simulink model "PositionControl"  (R2023a)
settings: Solver=FixedStepAuto  StartTime=0.0  StopTime=100.0  FixedStep=Ts  RelTol=1e-3
values from neighbouring files (symbols this model uses):
  refx = 5    [generar_circuito.m]    (also in generar_trayectoria.m = 1.3236)
  refy = 0    [generar_circuito.m]    (also in generar_trayectoria.m = -4.0246)
undefined symbols (not defined in the file or in its folder): DiscIntNeverNeededParam
libraries: fuzblock x1
settings Model: PacingRate=100  Creator=mfran  LastModifiedBy=mfran
settings DataIOCC: ReturnWorkspaceOutputs=off

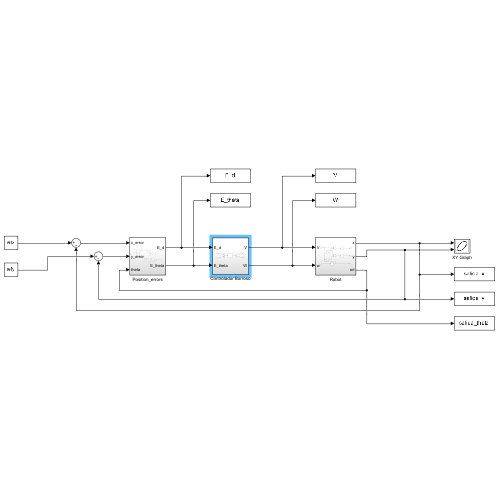
[thumbnail: Simulink's stored preview of the top-level diagram]
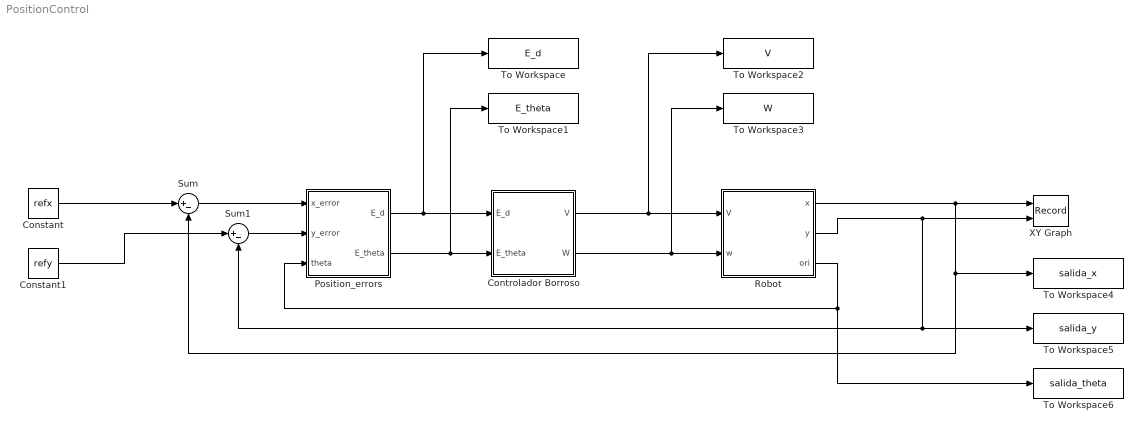
== system PositionControl ==
  Constant : Constant  Value=refx
  Constant1 : Constant  Value=refy
  Controlador Borroso : Subsystem
  Position_errors : Subsystem
  Robot : Subsystem
  Sum : Sum  Inputs=|+-
  Sum1 : Sum  Inputs=|+-
  To Workspace : ToWorkspace  VariableName=E_d  SaveFormat=Timeseries  SampleTime=-1
  To Workspace1 : ToWorkspace  VariableName=E_theta  SaveFormat=Timeseries  SampleTime=-1
  To Workspace2 : ToWorkspace  VariableName=V  SaveFormat=Timeseries  SampleTime=-1
  To Workspace3 : ToWorkspace  VariableName=W  SaveFormat=Timeseries  SampleTime=-1
  To Workspace4 : ToWorkspace  VariableName=salida_x  SaveFormat=Timeseries  SampleTime=-1
  To Workspace5 : ToWorkspace  VariableName=salida_y  SaveFormat=Timeseries  SampleTime=-1
  To Workspace6 : ToWorkspace  VariableName=salida_theta  SaveFormat=Timeseries  SampleTime=-1
  XY Graph : Record  FileSettingsInternal="{\"entries\":[{\"content\":{\"excelSettings\":{\"content\":{},\"type\":\"Streamout.ExcelSettings\"}},\"type\":\"Streamout.FileSettingStorage\",\"uuid\":\"\"}],\"packageUris\":[\"http:\\/\\/schema.mathworks.com\\/mf0\\/streamout_blocks\\/R2020a\"],\"version\":\"1.0\"}"  Layout=[1 1]  SignalsInternal="{\"entries\":[{\"content\":{\"signals\":[{\"content\":{\"blockPath\":[],\"dimensions\":[1],\"domain\":\"\",\"lineColor\":\"#a2142f\",\"plots\":[1],\"port\":1,\"sid\":[\"\"],\"signalID\":8169,\"signalName\":\"Robot:1\"},\"type\":\"RecordBlkView.Signal\",\"uuid\":\"\"},{\"content\":{\"blockPath\":[],\"dimensions\":[1],\"domain\":\"\",\"lineColor\":\"#139fff\",\"plots\":[1],\"port\":2,\"sid\":[\"\"],\"signalID\":8173,\"signalName\":\"Robot:2\"},\"type\":\"RecordBlkView.Signal\",\"uuid\":\"\"}]},\"type\":\"RecordBlkView.InputSignals\",\"uuid\":\"\"}],\"packageUris\":[\"http:\\/\\/schema.mathworks.com\\/mf0\\/streamout_blocks\\/R2020a\"],\"version\":\"1.0\"}"  VisualizationBindings="{\"xyplotplugin\":{\"info\":[{\"series\":[{\"bindingParametersList\":[{\"parameter\":\"X-Axis\",\"signalID\":8169,\"signalName\":\"Robot:1\"},{\"parameter\":\"Y-Axis\",\"signalID\":8173,\"signalName\":\"Robot:2\"}],\"seriesID\":46637}],\"subplotID\":1}]}}"  CompatibilityTag=XY
  wires:
  Controlador Borroso/1(V) -> To Workspace2/1, Robot/1(V)
  Controlador Borroso/2(W) -> To Workspace3/1, Robot/2(w)
  Position_errors/1(E_d) -> Controlador Borroso/1(E_d), To Workspace/1
  Position_errors/2(E_theta) -> Controlador Borroso/2(E_theta), To Workspace1/1
  Sum/1 -> Position_errors/1(x_error)
  Sum1/1 -> Position_errors/2(y_error)
  Robot/1(x) -> Sum/2, To Workspace4/1, XY Graph/1
  Robot/2(y) -> Sum1/2, To Workspace5/1, XY Graph/2
  Robot/3(ori) -> Position_errors/3(theta), To Workspace6/1
  Constant/1 -> Sum/1
  Constant1/1 -> Sum1/1

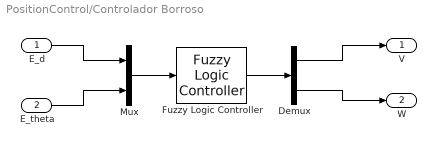
== system PositionControl/Controlador Borroso ==
  E_d : Inport
  E_theta : Inport  Port=2
  Demux : Demux  Outputs=2
  Fuzzy Logic Controller : fuzblock/Fuzzy Logic  Controller  FIS='FuzzyParteI.fis'  OutputSampleNumber=101  DataType=double  FuzzifiedInputs=off  RuleFiringStrengths=off  RuleOutputs=off  AggregatedOutputs=off  SimulateUsing=Interpreted execution  OutOfRangeInputValueMessage=warning  NoRuleFiredMessage=warning  EmptyOutputFuzzySetMessage=warning
  Mux : Mux  Inputs=2
  V : Outport
  W : Outport  Port=2
  wires:
  Demux/1 -> V/1
  Fuzzy Logic Controller/1 -> Demux/1
  Demux/2 -> W/1
  E_theta/1 -> Mux/2
  E_d/1 -> Mux/1
  Mux/1 -> Fuzzy Logic Controller/1

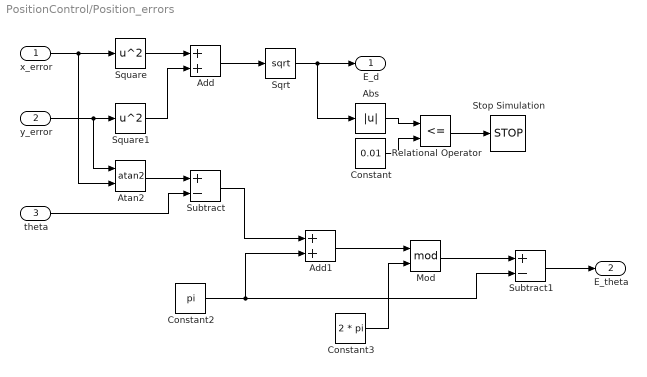
== system PositionControl/Position_errors ==
  x_error : Inport
  y_error : Inport  Port=2
  theta : Inport  Port=3
  Abs : Abs  SaturateOnIntegerOverflow=off
  Add : Sum
  Add1 : Sum
  Atan2 : Trigonometry  Operator=atan2
  Constant : Constant  Value=0.01
  Constant2 : Constant  Value=pi
  Constant3 : Constant  Value=2 * pi
  Mod : Math  Operator=mod
  Relational Operator : RelationalOperator  Operator=<=  OutDataTypeStr=boolean  RndMeth=Simplest  InputSameDT=off
  Sqrt : Sqrt
  Square : Math  Operator=square
  Square1 : Math  Operator=square
  Stop Simulation : Stop
  Subtract : Sum  Inputs=+-
  Subtract1 : Sum  Inputs=+-
  E_d : Outport
  E_theta : Outport  Port=2
  wires:
  Square1/1 -> Add/2
  Sqrt/1 -> Abs/1, E_d/1
  y_error/1 -> Atan2/1, Square1/1
  theta/1 -> Subtract/2
  x_error/1 -> Atan2/2, Square/1
  Atan2/1 -> Subtract/1
  Add/1 -> Sqrt/1
  Square/1 -> Add/1
  Abs/1 -> Relational Operator/1
  Constant/1 -> Relational Operator/2
  Relational Operator/1 -> Stop Simulation/1
  Mod/1 -> Subtract1/1
  Subtract/1 -> Add1/1
  Add1/1 -> Mod/1
  Constant2/1 -> Add1/2, Subtract1/2
  Constant3/1 -> Mod/2
  Subtract1/1 -> E_theta/1

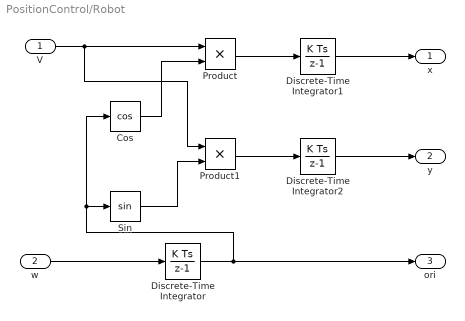
== system PositionControl/Robot ==
  V : Inport
  w : Inport  Port=2
  Cos : Trigonometry  Operator=cos
  Discrete-Time Integrator : DiscreteIntegrator  SampleTime=-1  ICPrevOutput=DiscIntNeverNeededParam  ICPrevScaledInput=DiscIntNeverNeededParam
  Discrete-Time Integrator1 : DiscreteIntegrator  SampleTime=-1  ICPrevOutput=DiscIntNeverNeededParam  ICPrevScaledInput=DiscIntNeverNeededParam
  Discrete-Time Integrator2 : DiscreteIntegrator  SampleTime=-1  ICPrevOutput=DiscIntNeverNeededParam  ICPrevScaledInput=DiscIntNeverNeededParam
  Product : Product
  Product1 : Product
  Sin : Trigonometry
  x : Outport
  y : Outport  Port=2
  ori : Outport  Port=3
  wires:
  Sin/1 -> Product1/2
  Discrete-Time Integrator1/1 -> x/1
  Discrete-Time Integrator2/1 -> y/1
  Product/1 -> Discrete-Time Integrator1/1
  V/1 -> Product1/1, Product/1
  Product1/1 -> Discrete-Time Integrator2/1
  Discrete-Time Integrator/1 -> ori/1, Sin/1, Cos/1
  w/1 -> Discrete-Time Integrator/1
  Cos/1 -> Product/2
